simulink model "vector"  (R2025b)
settings: Solver=FixedStepAuto  StartTime=0.0  StopTime=30  FixedStep=0.05  RelTol=1e-3
undefined symbols (not defined in the file or in its folder): DiscIntNeverNeededParam
libraries: rllib x1
(part 2 of 2)

== matlab function vector/Reward1/MATLAB Function ==
  data: cmd_vec input; e_v_dir output; velo input; e_v_mag output
function [e_v_dir, e_v_mag] = fcn(cmd_vec, velo)

    eps_val = 1e-6;

    cmd_vec = cmd_vec(:);
    velo    = velo(:);

    cmd_mag = norm(cmd_vec);
    vel_mag = norm(velo);

    % 1) 속도 크기 오차
    e_v_mag = abs(cmd_mag - vel_mag);

    % 2) 속도 방향 오차
    if (cmd_mag < eps_val) || (vel_mag < eps_val)
        e_v_dir = 0;
    else
        cmd_hat = cmd_vec / cmd_mag;
        vel_hat = velo / vel_mag;
        e_v_dir = 1 - dot(cmd_hat, vel_hat);
    end

end

== matlab function vector/Reward1/e_omega huber ==
  data: omega_error input; Loss_p output; Loss_q output; Loss_r output
function [Loss_p, Loss_q, Loss_r] = fcn(omega_error)

    p_error = omega_error(1);
    q_error = omega_error(2);
    r_error = omega_error(3);

    delta = 0.21;
    

    if abs(p_error) <= delta
        Loss_p = 0.5 * p_error^2;
    else
        Loss_p = delta * (abs(p_error) - 0.5 * delta);
    end

    if abs(q_error) <= delta
        Loss_q = 0.5 * q_error^2;
    else
        Loss_q = delta * (abs(q_error) - 0.5 * delta);
    end

    if abs(r_error) <= delta
        Loss_r = 0.5 * r_error^2;
    else
        Loss_r = delta * (abs(r_error) - 0.5 * delta);
    end

end

== matlab function vector/Reward1/e_pos huber ==
  data: pos_error input; Loss_x output; Loss_y output; Loss_z output
function [Loss_x, Loss_y, Loss_z] = fcn(pos_error)
    x_error = pos_error(1);
    y_error = pos_error(2);
    z_error = pos_error(3);

    horizon_delta = 0.21;
    vertical_delta = 0.029;

    if abs(x_error) <= horizon_delta
        Loss_x = 0.5 * x_error^2;
    else
        Loss_x = horizon_delta * (abs(x_error) - 0.5 * horizon_delta);
    end

    if abs(y_error) <= horizon_delta
        Loss_y = 0.5 * y_error^2;
    else
        Loss_y = horizon_delta * (abs(y_error) - 0.5 * horizon_delta);
    end

    if abs(z_error) <= vertical_delta
        Loss_z = 0.5 * z_error^2;
    else
        Loss_z = vertical_delta * (abs(z_error) - 0.5 * vertical_delta);
    end

end

== matlab function vector/Reward1/e_v_dir huber ==
  data: e_v_dir input; Loss_evdir output
function Loss_evdir = fcn(e_v_dir)

    delta = 0.003;
    e_v_dir = double(e_v_dir);
    e_v_dir = e_v_dir(1);   % scalar 보장

    if abs(e_v_dir) <= delta
        Loss_evdir = 0.5 * e_v_dir^2;
    else
        Loss_evdir = delta * (abs(e_v_dir) - 0.5 * delta);
    end

end

== matlab function vector/Reward1/e_v_mag huber ==
  data: e_v_mag input; Loss_evdir output
function Loss_evdir = fcn(e_v_mag)

    delta = 0.09;
    e_v_mag = double(e_v_mag);
    e_v_mag = e_v_mag(1);   % scalar 보장

    if abs(e_v_mag) <= delta
        Loss_evdir = 0.5 * e_v_mag^2;
    else
        Loss_evdir = delta * (abs(e_v_mag) - 0.5 * delta);
    end

end

== matlab function vector/Hybrid RL-PD Control System/MATLAB Function ==
  data: omega input; phidot output; att input; thetadot output; psidot output
function [phidot, thetadot, psidot] = Kinematics(omega, att)
    % omega = [p; q; r], att = [phi; theta; psi]
    phi = att(1); theta = att(2);
    
    % 오일러 각 변화율 계산 (좌표 변환)
    phidot   = omega(1) + sin(phi)*tan(theta)*omega(2) + cos(phi)*tan(theta)*omega(3);
    thetadot = cos(phi)*omega(2) - sin(phi)*omega(3);
    psidot   = (sin(phi)/cos(theta))*omega(2) + (cos(phi)/cos(theta))*omega(3);
end

== matlab function vector/Hybrid RL-PD Control System2/Attitude and Thrust Controller ==
  data: m input; g input; desired_acc input; U output; att input; omega input; max_thrust output
function [U, max_thrust] = fcn(m, g, desired_acc, att, omega)

    ax_des = desired_acc(1);
    ay_des = desired_acc(2);
    az_des = desired_acc(3);

    phi   = att(1);
    theta = att(2);
    psi   = att(3);

    p = omega(1); 
    q = omega(2);
    r = omega(3);

    psi_des = 0;

    max_tilt = deg2rad(30);
    max_thrust = 1.5 * m * g;
    min_thrust = 0;

    Kp_phi   = 7.0;   Kd_phi   = 0.9;
    Kp_theta = 7.0;   Kd_theta = 0.9;
    Kp_psi   = 0.5;   Kd_psi   = 0.2;

    phi_des   = ( ax_des*sin(psi) - ay_des*cos(psi) ) / g;
    theta_des = ( ax_des*cos(psi) + ay_des*sin(psi) ) / g;

    phi_des   = min(max(phi_des,   -max_tilt), max_tilt);
    theta_des = min(max(theta_des, -max_tilt), max_tilt);

    cphi = cos(phi);
    cth  = cos(theta);

    den = cphi * cth;
    den = max(den, 0.2);

    U1 = m * (g + az_des) / den;
    U1 = min(max(U1, min_thrust), max_thrust);

    e_phi   = phi_des - phi;
    e_theta = theta_des - theta;
    e_psi   = mod(psi_des - psi + pi, 2*pi) - pi;

    U2 = Kp_phi   * e_phi   - Kd_phi   * p;
    U3 = Kp_theta * e_theta - Kd_theta * q;
    U4 = Kp_psi   * e_psi   - Kd_psi   * r;

    U = [U1; U2; U3; U4];
end

== matlab function vector/Reward/e_v_mag huber ==
  data: e_v_mag input; Loss_evdir output; num input
function Loss_evdir = fcn(e_v_mag, num)

    delta = 0.12; % mode 1 기준
    % delta = 0.09; % mode 2 기준
    

    e_v_mag = double(e_v_mag);
    e_v_mag = e_v_mag(1);   % scalar 보장

    Loss_evdir = loss(delta, e_v_mag, num);

end

function L = loss(delta, error, num)

    if num == 1
        L = delta * abs(error);
    elseif num == 2
        L = 0.5 * error^2;
    else
        if abs(error) <= delta
            L = 0.5 * error^2;
        else
            L = delta * (abs(error) - 0.5 * delta);
        end
    end
end

== matlab function vector/Hybrid RL-PD Control System2/Commander ==
  data: select input; cmd_vec output; pos input; p_star output; B_pos input; R input
function [cmd_vec, p_star] = fcn(select, pos, B_pos, R)
    % 입력:
    %   select : 모드 선택
    %   pos    : 현재 위치 [x;y;z]
    %   B_pos  : 직선 비행 목표점
    %   R      : 원 반지름 / 8자 크기
    %
    % 출력:
    %   cmd_vec : 목표 속도 벡터 [vx; vy; vz]
    %   p_star  : 기준점(또는 목표점)

    pos = pos(:);
    B_pos = B_pos(:);

    cmd_vec = [0; 0; 0];
    p_star  = pos;

    v_max = 5;
    A_pos = [0; 0; 25];   % 기본 기준점

    % 8자 경로용 내부 파라미터
    persistent s_8;
    if isempty(s_8)
        s_8 = 0;
    end

    if select == 1   % 1) 제자리 호버링
        target_pos = A_pos;
        p_star = target_pos;

        e = target_pos - pos;
        d = norm(e);

        dir = e / (d + 1e-6);
        speed_cmd = v_max * tanh(0.6 * d);

        cmd_vec = speed_cmd * dir;

    elseif select == 2   % 2) A에서 B까지 이동 (직선)
        p_star = p_star_finder(A_pos, B_pos, pos);
        cmd_vec = line_vec_raw(A_pos, B_pos, pos);

    elseif select == 3   % 3) 원 비행
        z_ref = A_pos(3);
        C_pos = [A_pos(1) + R; A_pos(2); z_ref];
        [p_star, circle_dir] = circle_vec(C_pos, R, z_ref, pos);
        cmd_vec = v_max * circle_dir;

    elseif select == 4   % 4) 8자 비행 (carrot-chasing)

        % =========================================================
        % 설정
        % =========================================================
        A_8 = R;        % x 방향 크기
        B_8 = R / 2;    % y 방향 크기
        z_ref = A_pos(3);

        % 현재 가지(branch) 유지용 국소 탐색 창
        s_window = 0.08;    % 이전 s 주변 탐색 범위
        n_search = 60;      % 탐색 점 개수

        % 전방 목표점 look-ahead
        s_look = 0.04;      % 너무 작으면 흔들리고, 너무 크면 코너를 깎음

        % z 제어
        kz = 1.0;
        vz_max = 2.0;

        % =========================================================
        % 1) 이전 s_8 주변에서 국소 최근접점 탐색
        %    (전체 경로 탐색 X, 현재 가지 유지 목적)
        % =========================================================
        s_candidates = linspace(s_8 - s_window, s_8 + s_window, n_search);
        s_candidates = mod(s_candidates, 1.0);

        path_candidates = [A_pos(1) + A_8*sin(2*pi*s_candidates); ...
                           A_pos(2) + B_8*sin(4*pi*s_candidates); ...
                           z_ref * ones(1, n_search)];

        dists = sqrt(sum((path_candidates - pos).^2, 1));
        [~, idx_min] = min(dists);

        s_near = s_candidates(idx_min);

        % =========================================================
        % 2) 최근접점 p_star 계산
        % =========================================================
        p_star = [A_pos(1) + A_8*sin(2*pi*s_near); ...
                  A_pos(2) + B_8*sin(4*pi*s_near); ...
                  z_ref];

        % =========================================================
        % 3) look-ahead 목표점 p_target 계산
        % =========================================================
        s_target = mod(s_near + s_look, 1.0);

        p_target = [A_pos(1) + A_8*sin(2*pi*s_target); ...
                    A_pos(2) + B_8*sin(4*pi*s_target); ...
                    z_ref];

        % 다음 step을 위해 현재 진행률 저장
        s_8 = s_near;
        eps_val = 1e-6;
        e_xy = p_target(1:2) - pos(1:2);
        d_xy = norm(e_xy);

        v_xy = e_xy/(d_xy + eps_val);

        vz = kz * (z_ref - pos(3));
        v8 = [v_xy(1); v_xy(2); vz];
        v8_hat = v8/(norm(v8) + eps_val);
        

        cmd_vec = v_max*v8_hat; 

    else
        cmd_vec = [0; 0; 0];
        p_star  = pos;
        p_target = pos;
    end
end

== matlab function vector/Hybrid RL-PD Control System2/Drone Dynamics ==
  data: Th input; xddot output; att input; omega input; m input; g input; wind input; yddot output; zddot output; pdot output; qdot output; rdot output
function [xddot, yddot, zddot, pdot, qdot, rdot] = fcn(Th, att, omega, m, g, wind)
    assert(numel(Th) == 4);
    Th1 = Th(1);
    Th2 = Th(2);
    Th3 = Th(3);
    Th4 = Th(4);

    phi   = att(1);
    theta = att(2);
    psi   = att(3);

    p = omega(1);
    q = omega(2);
    r = omega(3);

    Fx = wind(1);
    Fy = wind(2);
    Fz = wind(3);

    l = 0.32;
    Ix = 0.07;
    Iy = 0.07;
    Iz = 0.12;
    kpsi = 0.05;

    U1 = Th1 + Th2 + Th3 + Th4;

    % Translational dynamics
    xddot = ( U1*(cos(psi)*sin(theta)*cos(phi) + sin(psi)*sin(phi)) + Fx ) / m;
    yddot = ( U1*(sin(psi)*sin(theta)*cos(phi) - cos(psi)*sin(phi)) + Fy ) / m;
    zddot = ( U1*(cos(theta)*cos(phi)) - m*g + Fz ) / m;

    % Torques
    tau_phi   = (l/sqrt(2)) * (Th1 - Th2 - Th3 + Th4);
    tau_theta = (l/sqrt(2)) * (Th1 + Th2 - Th3 - Th4);
    tau_psi   = kpsi*(-Th1 + Th2 - Th3 + Th4);

    % Euler angle kinematics
    cth = cos(theta);
    cth = sign(cth) * max(abs(cth), 1e-6);  % singularity guard

    phidot   = p + q*sin(phi)*tan(theta) + r*cos(phi)*tan(theta);
    thetadot = q*cos(phi) - r*sin(phi);
    psidot   = (q*sin(phi) + r*cos(phi)) / cth;

    % Rotational dynamics with coupling
    pdot = (tau_phi   + (Iy - Iz)*q*r) / Ix;
    qdot = (tau_theta + (Iz - Ix)*p*r) / Iy;
    rdot = (tau_psi   + (Ix - Iy)*p*q) / Iz;
end

== matlab function vector/Hybrid RL-PD Control System2/MATLAB Function ==
  data: omega input; phidot output; att input; thetadot output; psidot output
function [phidot, thetadot, psidot] = Kinematics(omega, att)
    % omega = [p; q; r], att = [phi; theta; psi]
    phi = att(1); theta = att(2);
    
    % 오일러 각 변화율 계산 (좌표 변환)
    phidot   = omega(1) + sin(phi)*tan(theta)*omega(2) + cos(phi)*tan(theta)*omega(3);
    thetadot = cos(phi)*omega(2) - sin(phi)*omega(3);
    psidot   = (sin(phi)/cos(theta))*omega(2) + (cos(phi)/cos(theta))*omega(3);
end

== matlab function vector/Hybrid RL-PD Control System2/Thrust Mixer ==
  data: U input; Th output; max_thrust input
function Th = fcn(U, max_thrust)

    U1 = U(1);
    U2 = U(2);
    U3 = U(3);
    U4 = U(4);

    l = 0.32;          % arm length [m]
    kpsi = 0.05;      % yaw mixing gain
    Th_max = max_thrust/4;

    a = sqrt(2)/(4*l);
    b = 1/(4*kpsi);
    
    Th1 = 0.25*U1 + a*U2 + a*U3 - b*U4;
    Th2 = 0.25*U1 - a*U2 + a*U3 + b*U4;
    Th3 = 0.25*U1 - a*U2 - a*U3 - b*U4;
    Th4 = 0.25*U1 + a*U2 - a*U3 + b*U4;

    Th1 = min(max(Th1, 0), Th_max);
    Th2 = min(max(Th2, 0), Th_max);
    Th3 = min(max(Th3, 0), Th_max);
    Th4 = min(max(Th4, 0), Th_max);

    Th = [Th1; Th2; Th3; Th4];

end

== matlab function vector/Hybrid RL-PD Control System2/Velocity-to-Acceleration Controller ==
  data: desired_acc output; cmd_vec input; vel input
% Velocity-to-Acceleration Controller
% 입력 -> 속도, 명령 벡터
% 출력 -> 가속도 벡터

function desired_acc = fcn(cmd_vec, vel)

    x_vel = vel(1);
    y_vel = vel(2);
    z_vel = vel(3);

    % x_error = pos_error(1);
    % y_error = pos_error(2);
    % z_error = pos_error(3);
    
    xv_error = cmd_vec(1) - x_vel;
    yv_error = cmd_vec(2) - y_vel;
    zv_error = cmd_vec(3) - z_vel;

    Kp_hoz = 4.4; 
    Kp_alt = 3; 

    desired_acc_x = Kp_hoz * xv_error;
    desired_acc_y = Kp_hoz * yv_error;
    desired_acc_z = Kp_alt * zv_error;

    desired_acc = [desired_acc_x; desired_acc_y; desired_acc_z];
    
end

== matlab function vector/Hybrid RL-PD Control System2/Wind/MATLAB Function3 ==
  data: seed input size=[1 1]; wind output
function wind = fcn(seed)
%#codegen
% seed : scalar double
% wind : [3x1] double

    % ===== 사용자 설정 =====
    Ts    = 0.01;
    tau   = [0.8; 0.8; 1.0];
    sigma = [1.0; 1.0; 0.5];
    clip  = 6.0;

    % ===== persistent states =====
    persistent w lastSeed n
    if isempty(w)
        w = zeros(3,1);
        lastSeed = -1;
        n = 0;
    end

    % ===== seed가 바뀌면 상태 리셋 =====
    if seed ~= lastSeed
        w = zeros(3,1);
        lastSeed = seed;
        n = 0;
    end

    % ===== OU update 계수 =====
    a = exp(-Ts ./ tau);
    b = sigma .* sqrt(max(0, 1 - a.^2));

    % ===== seed 기반 의사난수 생성 =====
    % 같은 seed면 같은 순서의 z가 나옴
    z = zeros(3,1);

    for k = 1:3
        t1 = seed*12.9898 + (n+1)*78.233 + k*37.719;
        t2 = seed*39.3467 + (n+1)*11.135 + k*83.155;

        u1 = sin(t1) * 43758.5453;
        u2 = sin(t2) * 24634.6345;

        u1 = u1 - floor(u1);   % frac(u1)
        u2 = u2 - floor(u2);   % frac(u2)

        % log(0) 방지
        if u1 < 1e-12
            u1 = 1e-12;
        end

        % Box-Muller
        z(k) = sqrt(-2.0*log(u1)) * cos(2.0*pi*u2);
    end

    % ===== 상태 업데이트 =====
    w = a .* w + b .* z;
    n = n + 1;

    % ===== saturation =====
    if isfinite(clip)
        w = min(max(w, -clip), clip);
    end

    wind = w;
end

== matlab function vector/Hybrid RL-PD Control System3/Attitude and Thrust Controller ==
  data: m input; g input; desired_acc input; U output; att input; omega input; max_thrust output
function [U, max_thrust] = fcn(m, g, desired_acc, att, omega)

    ax_des = desired_acc(1);
    ay_des = desired_acc(2);
    az_des = desired_acc(3);

    phi   = att(1);
    theta = att(2);
    psi   = att(3);

    p = omega(1); 
    q = omega(2);
    r = omega(3);

    psi_des = 0;

    max_tilt = deg2rad(30);
    max_thrust = 1.5 * m * g;
    min_thrust = 0;

    Kp_phi   = 15;   Kd_phi   = 2.5;
    Kp_theta = 15;   Kd_theta = 2.5;
    Kp_psi   = 0.5;   Kd_psi   = 0.2;

    phi_des   = ( ax_des*sin(psi) - ay_des*cos(psi) ) / g;
    theta_des = ( ax_des*cos(psi) + ay_des*sin(psi) ) / g;

    phi_des   = min(max(phi_des,   -max_tilt), max_tilt);
    theta_des = min(max(theta_des, -max_tilt), max_tilt);

    cphi = cos(phi);
    cth  = cos(theta);

    den = cphi * cth;
    den = max(den, 0.2);

    U1 = m * (g + az_des) / den;
    U1 = min(max(U1, min_thrust), max_thrust);

    e_phi   = phi_des - phi;
    e_theta = theta_des - theta;
    e_psi   = mod(psi_des - psi + pi, 2*pi) - pi;

    U2 = Kp_phi   * e_phi   - Kd_phi   * p;
    U3 = Kp_theta * e_theta - Kd_theta * q;
    U4 = Kp_psi   * e_psi   - Kd_psi   * r;

    U = [U1; U2; U3; U4];
end

== matlab function vector/Reward/e_pos huber ==
  data: pos_error input; Loss_x output; Loss_y output; Loss_z output; num input
function [Loss_x, Loss_y, Loss_z] = fcn(pos_error, num)
    x_error = pos_error(1);
    y_error = pos_error(2);
    z_error = pos_error(3);

    % horizon_delta = 0.048;
    % vertical_delta = 0.018;

    x_delta = 0.070;
    % y_delta = 0.066;
    z_delta = 0.02;
    
    % x_delta = 0.037`
    % y_delta = 0.091;
    % z_delta = 0.043;

    Loss_x = loss(x_delta, x_error, num);
    Loss_y = loss(x_delta, y_error, num);
    Loss_z = loss(z_delta, z_error, num);
end

function L = loss(delta, error, num)

    if num == 1
        L = delta * abs(error);
    elseif num == 2
        L = 0.5 * error^2;
    else
        if abs(error) <= delta
            L = 0.5 * error^2;
        else
            L = delta * (abs(error) - 0.5 * delta);
        end
    end
end

== matlab function vector/Hybrid RL-PD Control System3/Commander ==
  data: select input; cmd_vec output; pos input; p_star output; B_pos input; R input
function [cmd_vec, p_star] = fcn(select, pos, B_pos, R)
    % 입력:
    %   select : 모드 선택
    %   pos    : 현재 위치 [x;y;z]
    %   B_pos  : 직선 비행 목표점
    %   R      : 원 반지름 / 8자 크기
    %
    % 출력:
    %   cmd_vec : 목표 속도 벡터 [vx; vy; vz]
    %   p_star  : 기준점(또는 목표점)

    pos = pos(:);
    B_pos = B_pos(:);

    cmd_vec = [0; 0; 0];
    p_star  = pos;

    v_max = 5;
    A_pos = [0; 0; 25];   % 기본 기준점

    % 8자 경로용 내부 파라미터
    persistent s_8;
    if isempty(s_8)
        s_8 = 0;
    end

    if select == 1 % 1) 제자리 호버링 
        target_pos = A_pos; 
        p_star = target_pos; 
        e = target_pos - pos; d = norm(e); 
        dir = e / (d + 1e-6); 
        speed_cmd = v_max * tanh(0.6 * d); 
        cmd_vec = speed_cmd * dir;
        
    elseif select == 2   % 2) A에서 B까지 이동 (직선)
        p_star = p_star_finder(A_pos, B_pos, pos);
        cmd_vec = line_vec_raw(A_pos, B_pos, pos);

    elseif select == 3   % 3) 원 비행
        z_ref = A_pos(3);
        C_pos = [A_pos(1) + R; A_pos(2); z_ref];
        [p_star, circle_dir] = circle_vec(C_pos, R, z_ref, pos);
        cmd_vec = v_max * circle_dir;

    elseif select == 4   % 4) 8자 비행 (carrot-chasing)

        % =========================================================
        % 설정
        % =========================================================
        A_8 = R;        % x 방향 크기
        B_8 = R / 2;    % y 방향 크기
        z_ref = A_pos(3);

        % 현재 가지(branch) 유지용 국소 탐색 창
        s_window = 0.08;    % 이전 s 주변 탐색 범위
        n_search = 60;      % 탐색 점 개수

        % 전방 목표점 look-ahead
        s_look = 0.04;      % 너무 작으면 흔들리고, 너무 크면 코너를 깎음

        % z 제어
        kz = 1.0;
        vz_max = 2.0;

        % =========================================================
        % 1) 이전 s_8 주변에서 국소 최근접점 탐색
        %    (전체 경로 탐색 X, 현재 가지 유지 목적)
        % =========================================================
        s_candidates = linspace(s_8 - s_window, s_8 + s_window, n_search);
        s_candidates = mod(s_candidates, 1.0);

        path_candidates = [A_pos(1) + A_8*sin(2*pi*s_candidates); ...
                           A_pos(2) + B_8*sin(4*pi*s_candidates); ...
                           z_ref * ones(1, n_search)];

        dists = sqrt(sum((path_candidates - pos).^2, 1));
        [~, idx_min] = min(dists);

        s_near = s_candidates(idx_min);

        % =========================================================
        % 2) 최근접점 p_star 계산
        % =========================================================
        p_star = [A_pos(1) + A_8*sin(2*pi*s_near); ...
                  A_pos(2) + B_8*sin(4*pi*s_near); ...
                  z_ref];

        % =========================================================
        % 3) look-ahead 목표점 p_target 계산
        % =========================================================
        s_target = mod(s_near + s_look, 1.0);

        p_target = [A_pos(1) + A_8*sin(2*pi*s_target); ...
                    A_pos(2) + B_8*sin(4*pi*s_target); ...
                    z_ref];

        % 다음 step을 위해 현재 진행률 저장
        s_8 = s_near;
        eps_val = 1e-6;
        e_xy = p_target(1:2) - pos(1:2);
        d_xy = norm(e_xy);

        v_xy = e_xy/(d_xy + eps_val);

        vz = kz * (z_ref - pos(3));
        v8 = [v_xy(1); v_xy(2); vz];
        v8_hat = v8/(norm(v8) + eps_val);
        

        cmd_vec = v_max*v8_hat; 

    else
        cmd_vec = [0; 0; 0];
        p_star  = pos;
        p_target = pos;
    end
end

== matlab function vector/Hybrid RL-PD Control System3/Subsystem/Drone Dynamics ==
  data: Th input; xddot output; att input; omega input; m input; g input; wind input; yddot output; zddot output; pdot output; qdot output; rdot output
function [xddot, yddot, zddot, pdot, qdot, rdot] = fcn(Th, att, omega, m, g, wind)
    assert(numel(Th) == 4);
    Th1 = Th(1);
    Th2 = Th(2);
    Th3 = Th(3);
    Th4 = Th(4);

    phi   = att(1);
    theta = att(2);
    psi   = att(3);

    p = omega(1);
    q = omega(2);
    r = omega(3);

    Fx = wind(1);
    Fy = wind(2);
    Fz = wind(3);

    l = 0.32;
    Ix = 0.07;
    Iy = 0.07;
    Iz = 0.12;
    kpsi = 0.05;

    U1 = Th1 + Th2 + Th3 + Th4;

    % Translational dynamics
    xddot = ( U1*(cos(psi)*sin(theta)*cos(phi) + sin(psi)*sin(phi)) + Fx ) / m;
    yddot = ( U1*(sin(psi)*sin(theta)*cos(phi) - cos(psi)*sin(phi)) + Fy ) / m;
    zddot = ( U1*(cos(theta)*cos(phi)) - m*g + Fz ) / m;

    % Torques
    tau_phi   = (l/sqrt(2)) * (Th1 - Th2 - Th3 + Th4);
    tau_theta = (l/sqrt(2)) * (Th1 + Th2 - Th3 - Th4);
    tau_psi   = kpsi*(-Th1 + Th2 - Th3 + Th4);

    % Euler angle kinematics
    cth = cos(theta);
    cth = sign(cth) * max(abs(cth), 1e-6);  % singularity guard

    % phidot   = p + q*sin(phi)*tan(theta) + r*cos(phi)*tan(theta);
    % thetadot = q*cos(phi) - r*sin(phi);
    % psidot   = (q*sin(phi) + r*cos(phi)) / cth;

    % Rotational dynamics with coupling
    pdot = (tau_phi   + (Iy - Iz)*q*r) / Ix;
    qdot = (tau_theta + (Iz - Ix)*p*r) / Iy;
    rdot = (tau_psi   + (Ix - Iy)*p*q) / Iz;
end

== matlab function vector/Hybrid RL-PD Control System3/Subsystem/MATLAB Function ==
  data: omega input; phidot output; att input; thetadot output; psidot output
function [phidot, thetadot, psidot] = Kinematics(omega, att)
    % omega = [p; q; r], att = [phi; theta; psi]
    phi = att(1); theta = att(2);
    
    % 오일러 각 변화율 계산 (좌표 변환)
    phidot   = omega(1) + sin(phi)*tan(theta)*omega(2) + cos(phi)*tan(theta)*omega(3);
    thetadot = cos(phi)*omega(2) - sin(phi)*omega(3);
    psidot   = (sin(phi)/cos(theta))*omega(2) + (cos(phi)/cos(theta))*omega(3);
end

== matlab function vector/Hybrid RL-PD Control System3/Thrust Mixer ==
  data: U input; Th output; max_thrust input
function Th = fcn(U, max_thrust)

    U1 = U(1);
    U2 = U(2);
    U3 = U(3);
    U4 = U(4);

    l = 0.32;          % arm length [m]
    kpsi = 0.05;      % yaw mixing gain
    Th_max = max_thrust/4;

    a = sqrt(2)/(4*l);
    b = 1/(4*kpsi);
    
    Th1 = 0.25*U1 + a*U2 + a*U3 - b*U4;
    Th2 = 0.25*U1 - a*U2 + a*U3 + b*U4;
    Th3 = 0.25*U1 - a*U2 - a*U3 - b*U4;
    Th4 = 0.25*U1 + a*U2 - a*U3 + b*U4;

    Th1 = min(max(Th1, 0), Th_max);
    Th2 = min(max(Th2, 0), Th_max);
    Th3 = min(max(Th3, 0), Th_max);
    Th4 = min(max(Th4, 0), Th_max);

    Th = [Th1; Th2; Th3; Th4];

end

== matlab function vector/Hybrid RL-PD Control System3/Velocity-to-Acceleration Controller ==
  data: desired_acc output; cmd_vec input; vel input
% Velocity-to-Acceleration Controller
% 입력 -> 속도, 명령 벡터
% 출력 -> 가속도 벡터

function desired_acc = fcn(cmd_vec, vel)

    x_vel = vel(1);
    y_vel = vel(2);
    z_vel = vel(3);

    % x_error = pos_error(1);
    % y_error = pos_error(2);
    % z_error = pos_error(3);
    
    xv_error = cmd_vec(1) - x_vel;
    yv_error = cmd_vec(2) - y_vel;
    zv_error = cmd_vec(3) - z_vel;

    Kp_hoz = 4.5; 
    Kp_alt = 3; 

    desired_acc_x = Kp_hoz * xv_error;
    desired_acc_y = Kp_hoz * yv_error;
    desired_acc_z = Kp_alt * zv_error;

    desired_acc = [desired_acc_x; desired_acc_y; desired_acc_z];
    
end

== matlab function vector/Hybrid RL-PD Control System3/Wind Subsystem/Wind/MATLAB Function3 ==
  data: seed input size=[1 1]; wind output
function wind = fcn(seed)
%#codegen
% seed : scalar double
% wind : [3x1] double

    % ===== 사용자 설정 =====
    Ts    = 0.01;
    tau   = [0.8; 0.8; 1.0];
    sigma = [1.0; 1.0; 0.5];
    clip  = 6.0;

    % ===== persistent states =====
    persistent w lastSeed n
    if isempty(w)
        w = zeros(3,1);
        lastSeed = -1;
        n = 0;
    end

    % ===== seed가 바뀌면 상태 리셋 =====
    if seed ~= lastSeed
        w = zeros(3,1);
        lastSeed = seed;
        n = 0;
    end

    % ===== OU update 계수 =====
    a = exp(-Ts ./ tau);
    b = sigma .* sqrt(max(0, 1 - a.^2));

    % ===== seed 기반 의사난수 생성 =====
    % 같은 seed면 같은 순서의 z가 나옴
    z = zeros(3,1);

    for k = 1:3
        t1 = seed*12.9898 + (n+1)*78.233 + k*37.719;
        t2 = seed*39.3467 + (n+1)*11.135 + k*83.155;

        u1 = sin(t1) * 43758.5453;
        u2 = sin(t2) * 24634.6345;

        u1 = u1 - floor(u1);   % frac(u1)
        u2 = u2 - floor(u2);   % frac(u2)

        % log(0) 방지
        if u1 < 1e-12
            u1 = 1e-12;
        end

        % Box-Muller
        z(k) = sqrt(-2.0*log(u1)) * cos(2.0*pi*u2);
    end

    % ===== 상태 업데이트 =====
    w = a .* w + b .* z;
    n = n + 1;

    % ===== saturation =====
    if isfinite(clip)
        w = min(max(w, -clip), clip);
    end

    wind = w;
end

== matlab function vector/Reward2/ e_angle huber ==
  data: angle_error input; Loss_phi output; Loss_theta output; Loss_psi output
function [Loss_phi, Loss_theta, Loss_psi] = fcn(angle_error)

    phi_error = angle_error(1);
    theta_error = angle_error(2);
    psi_error = mod(angle_error(3) + pi, 2*pi) - pi;

    % delta = 0.08; % mode 1 기준
    delta = 0.08; % mode 2 기준

    if abs(phi_error) <= delta
        Loss_phi = 0.5 * phi_error^2;
    else
        Loss_phi = delta * (abs(phi_error) - 0.5 * delta);
    end

    if abs(theta_error) <= delta
        Loss_theta = 0.5 * theta_error^2;
    else
        Loss_theta = delta * (abs(theta_error) - 0.5 * delta);
    end

    if abs(psi_error) <= delta
        Loss_psi = 0.5 * psi_error^2;
    else
        Loss_psi = delta * (abs(psi_error) - 0.5 * delta);
    end

end

== matlab function vector/Reward2/MATLAB Function ==
  data: cmd_vec input; e_v_dir output; velo input; e_v_mag output
function [e_v_dir, e_v_mag] = fcn(cmd_vec, velo)

    eps_val = 1e-6;

    cmd_vec = cmd_vec(:);
    velo    = velo(:);

    cmd_mag = norm(cmd_vec);
    vel_mag = norm(velo);

    % 1) 속도 크기 오차
    e_v_mag = abs(cmd_mag - vel_mag);

    % 2) smooth normalized vectors
    cmd_hat = cmd_vec / sqrt(cmd_mag^2 + eps_val^2);
    vel_hat = velo    / sqrt(vel_mag^2 + eps_val^2);

    c = dot(cmd_hat, vel_hat);
    c = max(-1, min(1, c));

    % 기본 방향 오차
    dir_raw = 1 - c;

    % 작은 속도에서는 방향 의미를 줄이는 smooth weight
    w = (cmd_mag * vel_mag) / ((cmd_mag * vel_mag) + eps_val^2);

    e_v_dir = w * dir_raw;

end

== matlab function vector/Reward2/e_omega huber ==
  data: omega_error input; Loss_p output; Loss_q output; Loss_r output
function [Loss_p, Loss_q, Loss_r] = fcn(omega_error)

    p_error = omega_error(1);
    q_error = omega_error(2);
    r_error = omega_error(3);

    % delta = 0.24; % mode 1 기준
    delta = 0.15; % mode 2 기준
    

    if abs(p_error) <= delta
        Loss_p = 0.5 * p_error^2;
    else
        Loss_p = delta * (abs(p_error) - 0.5 * delta);
    end

    if abs(q_error) <= delta
        Loss_q = 0.5 * q_error^2;
    else
        Loss_q = delta * (abs(q_error) - 0.5 * delta);
    end

    if abs(r_error) <= delta
        Loss_r = 0.5 * r_error^2;
    else
        Loss_r = delta * (abs(r_error) - 0.5 * delta);
    end

end

== matlab function vector/Reward2/e_pos huber ==
  data: pos_error input; Loss_x output; Loss_y output; Loss_z output
function [Loss_x, Loss_y, Loss_z] = fcn(pos_error)
    x_error = pos_error(1);
    y_error = pos_error(2);
    z_error = pos_error(3);

    % horizon_delta = 0.048;
    % vertical_delta = 0.018;

    x_delta = 0.037;
    y_delta = 0.091;
    z_delta = 0.043;

    if abs(x_error) <= x_delta
        Loss_x = 0.5 * x_error^2;
    else
        Loss_x = x_delta * (abs(x_error) - 0.5 * x_delta);
    end

    if abs(y_error) <= y_delta
        Loss_y = 0.5 * y_error^2;
    else
        Loss_y = y_delta * (abs(y_error) - 0.5 * y_delta);
    end

    if abs(z_error) <= z_delta
        Loss_z = 0.5 * z_error^2;
    else
        Loss_z = z_delta * (abs(z_error) - 0.5 * z_delta);
    end

end

== matlab function vector/Reward2/e_v_dir huber ==
  data: e_v_dir input; Loss_evdir output
function Loss_evdir = fcn(e_v_dir)

    % delta = 1.2; % mode 1 기준
    delta = 0.53; % mode 2 기준
    e_v_dir = double(e_v_dir);
    e_v_dir = e_v_dir(1);   % scalar 보장

    if abs(e_v_dir) <= delta
        Loss_evdir = 0.5 * e_v_dir^2;
    else
        Loss_evdir = delta * (abs(e_v_dir) - 0.5 * delta);
    end

end

== matlab function vector/Reward/ e_angle huber ==
  data: angle_error input; Loss_phi output; Loss_theta output; Loss_psi output; num input
function [Loss_phi, Loss_theta, Loss_psi] = fcn(angle_error, num)

    phi_error = angle_error(1);
    theta_error = angle_error(2);
    psi_error = mod(angle_error(3) + pi, 2*pi) - pi;

    delta = 0.12; % mode 1 기준
    % delta = 0.08; % mode 2 기준

    Loss_phi = loss(delta, phi_error, num);
    Loss_theta = loss(delta, theta_error, num);
    Loss_psi = loss(delta, psi_error, num);

end

function L = loss(delta, error, num)

    if num == 1
        L = delta * abs(error);
    elseif num == 2
        L = 0.5 * error^2;
    else
        if abs(error) <= delta
            L = 0.5 * error^2;
        else
            L = delta * (abs(error) - 0.5 * delta);
        end
    end
end

== matlab function vector/Reward2/e_v_mag huber ==
  data: e_v_mag input; Loss_evdir output
function Loss_evdir = fcn(e_v_mag)

    % delta = 0.075; % mode 1 기준
    delta = 0.09; % mode 2 기준
    

    e_v_mag = double(e_v_mag);
    e_v_mag = e_v_mag(1);   % scalar 보장

    if abs(e_v_mag) <= delta
        Loss_evdir = 0.5 * e_v_mag^2;
    else
        Loss_evdir = delta * (abs(e_v_mag) - 0.5 * delta);
    end

end

== matlab function vector/Hybrid RL-PD Control System/MATLAB Function1 ==
  data: percent input; u input; u_sat output; m input; g input
function u_sat = sat_agent_thrust(percent, u, m, g)

%#codegen

    Thrust_limit = 1.5 * m * g;
    
    upper =  percent * Thrust_limit;
    lower = -percent * Thrust_limit;
    
    u_sat = min(max(u, lower), upper);

end

== matlab function vector/Hybrid RL-PD Control System/Wind/Sine Wave ==
  data: seed input size=[1 1]; wind output
function wind = fcn(seed)
%#codegen
% seed : scalar double
% wind : [3x1] double, [Fx; Fy; Fz]
%
% Seeded multi-harmonic sine wind disturbance
% Each axis consists of fundamental + 3rd + 5th + 7th harmonic
% with fixed amplitudes and seed-dependent random phases.

    % =========================================================
    % 1) User settings
    % =========================================================
    Ts = 0.05;          % sampling time [s]
    f0 = 0.20;          % fundamental frequency [Hz]
    w0 = 2.0*pi*f0;     % fundamental angular frequency [rad/s]

    % Amplitudes for [fundamental, 3rd, 5th, 7th harmonic]
    % Rows: x, y, z axes
    % Fx, Fy max theoretical sum = 3 + 1.5 + 1 + 0.5 = 6
    % Fz max theoretical sum     = 1.5 + 0.75 + 0.5 + 0.25 = 3
    A = [ ...
        3.0, 1.5, 1.0, 0.5; ...
        3.0, 1.5, 1.0, 0.5; ...
        1.5, 0.75, 0.5, 0.25];

    clip = 6.0;         % saturation bound for each axis

    % Harmonic multipliers: fundamental, 3rd, 5th, 7th harmonic
    h = [1.0; 3.0; 5.0; 7.0];

    % =========================================================
    % 2) Persistent states
    % =========================================================
    persistent phase lastSeed n

    if isempty(phase)
        phase = zeros(3,4);    % rows: x,y,z / cols: 1st,3rd,5th,7th
        lastSeed = -1;
        n = 0;
    end

    % =========================================================
    % 3) Regenerate phases only when seed changes
    % =========================================================
    if seed ~= lastSeed
        phase = zeros(3,4);

        for axisIdx = 1:3
            for harmIdx = 1:4
                % Deterministic pseudo-random number in [0,1)
                s = seed*12.9898 ...
                    + axisIdx*78.233 ...
                    + harmIdx*37.719;

                u = sin(s) * 43758.5453;
                u = u - floor(u);   % frac(u)

                % Random phase in [0, 2*pi)
                phase(axisIdx, harmIdx) = 2.0*pi*u;
            end
        end

        lastSeed = seed;
        n = 0;
    end

    % =========================================================
    % 4) Generate multi-harmonic sine wind
    % =========================================================
    t = n * Ts;
    wind = zeros(3,1);

    for axisIdx = 1:3
        F = 0.0;

        for harmIdx = 1:4
            F = F + A(axisIdx, harmIdx) * ...
                sin(h(harmIdx)*w0*t + phase(axisIdx, harmIdx));
        end

        wind(axisIdx) = F;
    end

    n = n + 1;

    % =========================================================
    % 5) Saturation
    % =========================================================
    if isfinite(clip)
        wind = min(max(wind, -clip), clip);
    end
end

== matlab function vector/Reward/e_omega huber ==
  data: omega_error input; Loss_p output; Loss_q output; Loss_r output; num input
function [Loss_p, Loss_q, Loss_r] = fcn(omega_error, num)

    p_error = omega_error(1);
    q_error = omega_error(2);
    r_error = omega_error(3);

    delta = 0.53; % mode 1 기준
    % delta = 0.15; % mode 2 기준
    delta_r = 0.027;
    

    Loss_p = loss(delta, p_error, num);
    Loss_q = loss(delta, q_error, num);
    Loss_r = loss(delta_r, r_error, num);

end

function L = loss(delta, error, num)

    if num == 1
        L = delta * abs(error);
    elseif num == 2
        L = 0.5 * error^2;
    else
        if abs(error) <= delta
            L = 0.5 * error^2;
        else
            L = delta * (abs(error) - 0.5 * delta);
        end
    end
end

== matlab function vector/Hybrid RL-PD Control System/Velocity-to-Acceleration Controller ==
  data: desired_acc output; cmd_vec input; vel input
% Velocity-to-Acceleration Controller
% 입력 -> 속도, 명령 벡터
% 출력 -> 가속도 벡터

function desired_acc = fcn(cmd_vec, vel)

    x_vel = vel(1);
    y_vel = vel(2);
    z_vel = vel(3);

    % x_error = pos_error(1);
    % y_error = pos_error(2);
    % z_error = pos_error(3);
    
    xv_error = cmd_vec(1) - x_vel;
    yv_error = cmd_vec(2) - y_vel;
    zv_error = cmd_vec(3) - z_vel;

    Kp_hoz = 4.5; 
    Kp_alt = 3; 

    desired_acc_x = Kp_hoz * xv_error;
    desired_acc_y = Kp_hoz * yv_error;
    desired_acc_z = Kp_alt * zv_error;

    desired_acc = [desired_acc_x; desired_acc_y; desired_acc_z];
    
end

== matlab function vector/Hybrid RL-PD Control System/Attitude and Thrust Controller ==
  data: m input; g input; desired_acc input; U output; att input; omega input; max_thrust output
function [U, max_thrust] = fcn(m, g, desired_acc, att, omega)

    ax_des = desired_acc(1);
    ay_des = desired_acc(2);
    az_des = desired_acc(3);

    phi   = att(1);
    theta = att(2);
    psi   = att(3);

    p = omega(1); 
    q = omega(2);
    r = omega(3);

    psi_des = 0;

    max_tilt = deg2rad(30);
    max_thrust = 1.5 * m * g;
    min_thrust = 0;

    Kp_phi   = 15;   Kd_phi   = 2.5;
    Kp_theta = 15;   Kd_theta = 2.5;
    Kp_psi   = 0.5;   Kd_psi   = 0.2;

    phi_des   = ( ax_des*sin(psi) - ay_des*cos(psi) ) / g;
    theta_des = ( ax_des*cos(psi) + ay_des*sin(psi) ) / g;

    phi_des   = min(max(phi_des,   -max_tilt), max_tilt);
    theta_des = min(max(theta_des, -max_tilt), max_tilt);

    cphi = cos(phi);
    cth  = cos(theta);

    den = cphi * cth;
    den = max(den, 0.2);

    U1 = m * (g + az_des) / den;
    U1 = min(max(U1, min_thrust), max_thrust);

    e_phi   = phi_des - phi;
    e_theta = theta_des - theta;
    e_psi   = mod(psi_des - psi + pi, 2*pi) - pi;

    U2 = Kp_phi   * e_phi   - Kd_phi   * p;
    U3 = Kp_theta * e_theta - Kd_theta * q;
    U4 = Kp_psi   * e_psi   - Kd_psi   * r;

    U = [U1; U2; U3; U4];
end

== matlab function vector/Hybrid RL-PD Control System/Thrust Mixer ==
  data: U input; Th output; max_thrust input
function Th = fcn(U, max_thrust)

    U1 = U(1);
    U2 = U(2);
    U3 = U(3);
    U4 = U(4);

    l = 0.32;          % arm length [m]
    kpsi = 0.05;      % yaw mixing gain
    Th_max = max_thrust/4;

    a = sqrt(2)/(4*l);
    b = 1/(4*kpsi);
    
    Th1 = 0.25*U1 + a*U2 + a*U3 - b*U4;
    Th2 = 0.25*U1 - a*U2 + a*U3 + b*U4;
    Th3 = 0.25*U1 - a*U2 - a*U3 - b*U4;
    Th4 = 0.25*U1 + a*U2 - a*U3 + b*U4;

    Th1 = min(max(Th1, 0), Th_max);
    Th2 = min(max(Th2, 0), Th_max);
    Th3 = min(max(Th3, 0), Th_max);
    Th4 = min(max(Th4, 0), Th_max);

    Th = [Th1; Th2; Th3; Th4];

end

== matlab function vector/Hybrid RL-PD Control System/Drone Dynamics ==
  data: Th input; xddot output; att input; omega input; m input; g input; wind input; yddot output; zddot output; pdot output; qdot output; rdot output
function [xddot, yddot, zddot, pdot, qdot, rdot] = fcn(Th, att, omega, m, g, wind)
    assert(numel(Th) == 4);
    Th1 = Th(1);
    Th2 = Th(2);
    Th3 = Th(3);
    Th4 = Th(4);

    phi   = att(1);
    theta = att(2);
    psi   = att(3);

    p = omega(1);
    q = omega(2);
    r = omega(3);

    Fx = wind(1);
    Fy = wind(2);
    Fz = wind(3);

    l = 0.32;
    Ix = 0.07;
    Iy = 0.07;
    Iz = 0.12;
    kpsi = 0.05;

    U1 = Th1 + Th2 + Th3 + Th4;

    % Translational dynamics
    xddot = ( U1*(cos(psi)*sin(theta)*cos(phi) + sin(psi)*sin(phi)) + Fx ) / m;
    yddot = ( U1*(sin(psi)*sin(theta)*cos(phi) - cos(psi)*sin(phi)) + Fy ) / m;
    zddot = ( U1*(cos(theta)*cos(phi)) - m*g + Fz ) / m;

    % Torques
    tau_phi   = (l/sqrt(2)) * (Th1 - Th2 - Th3 + Th4);
    tau_theta = (l/sqrt(2)) * (Th1 + Th2 - Th3 - Th4);
    tau_psi   = kpsi*(-Th1 + Th2 - Th3 + Th4);

    % Euler angle kinematics
    cth = cos(theta);
    cth = sign(cth) * max(abs(cth), 1e-6);  % singularity guard

    % phidot   = p + q*sin(phi)*tan(theta) + r*cos(phi)*tan(theta);
    % thetadot = q*cos(phi) - r*sin(phi);
    % psidot   = (q*sin(phi) + r*cos(phi)) / cth;

    % Rotational dynamics with coupling
    pdot = (tau_phi   + (Iy - Iz)*q*r) / Ix;
    qdot = (tau_theta + (Iz - Ix)*p*r) / Iy;
    rdot = (tau_psi   + (Ix - Iy)*p*q) / Iz;
end
